simulink model "que3"  (R2015a)
settings: Solver=ode45  StartTime=0  StopTime=10.0  RelTol=1e-3
libraries: simulink x1
settings Model: Creator=Student  LastModifiedBy=Student

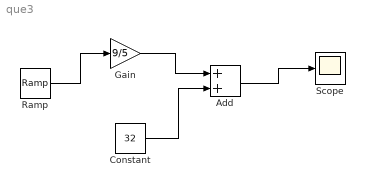
== system que3 ==
  Add : Sum
  Constant : Constant  Value=32
  Gain : Gain  Gain=9/5
  Ramp : simulink/Sources/Ramp  slope=1  start=0  X0=0
  Scope : Scope
  wires:
  Ramp/1 -> Gain/1
  Add/1 -> Scope/1
  Gain/1 -> Add/1
  Constant/1 -> Add/2
